simulink model "uc3_preparation1_2017"  (R2018a)
settings: Solver=FixedStepDiscrete  StartTime=0.0  StopTime=0.6  FixedStep=2e-5  RelTol=1e-3
libraries: simulink x10, hdlsllib x10, dspswit3 x1
(part 1 of 2)
settings Model: Creator=elahifah16  LastModifiedBy=Talha Rao
settings OptimizationCC: DefaultParameterBehavior=Inlined  DefaultUnderspecifiedDataType=single  PassReuseOutputArgsAs=Individual arguments
settings DebuggingCC: ParameterTunabilityLossMsg=error  BusObjectLabelMismatch=error
settings HardwareCC: ProdBitPerPointer=32  ProdBitPerSizeT=32  ProdBitPerPtrDiffT=32  ProdLargestAtomicInteger=Long  ProdLargestAtomicFloat=Double  ProdIntDivRoundTo=Undefined  ProdEndianess=Unspecified  ProdWordSize=32  ProdHWDeviceType=ARM Compatible->ARM Cortex
settings SFSimCC: MATLABDynamicMemAlloc=off
settings RTWCC: SystemTargetFile=ert.tlc  GenCodeOnly=on  TemplateMakefile=ert_default_tmf  GenerateReport=on  IncludeHyperlinkInReport=on  LaunchReport=on  GenerateTraceInfo=on  GenerateTraceReport=on  GenerateTraceReportSl=on  GenerateTraceReportSf=on  GenerateTraceReportEml=on  GenerateCodeReplacementReport=on
settings CodeAppCC: ForceParamTrailComments=on  IgnoreCustomStorageClasses=off  OperatorAnnotations=on  SimulinkDataObjDesc=on  SFDataObjDesc=on  InsertBlockDesc=on  StateflowObjectComments=on
settings ERTTargetCC: TargetLangStandard=C99 (ISO)  CodeReplacementLibrary=GNU C99 extensions  GenerateSampleERTMain=on  SupportComplex=off  SupportVariableSizeSignals=on  ExtModeTransport=1  ExtModeMexFile=ext_serial_win32_comm  InlinedParameterPlacement=NonHierarchical  MultiInstanceErrorCode=None  RootIOFormat=Structure reference  ERTCustomFileTemplate=example_file_process.tlc

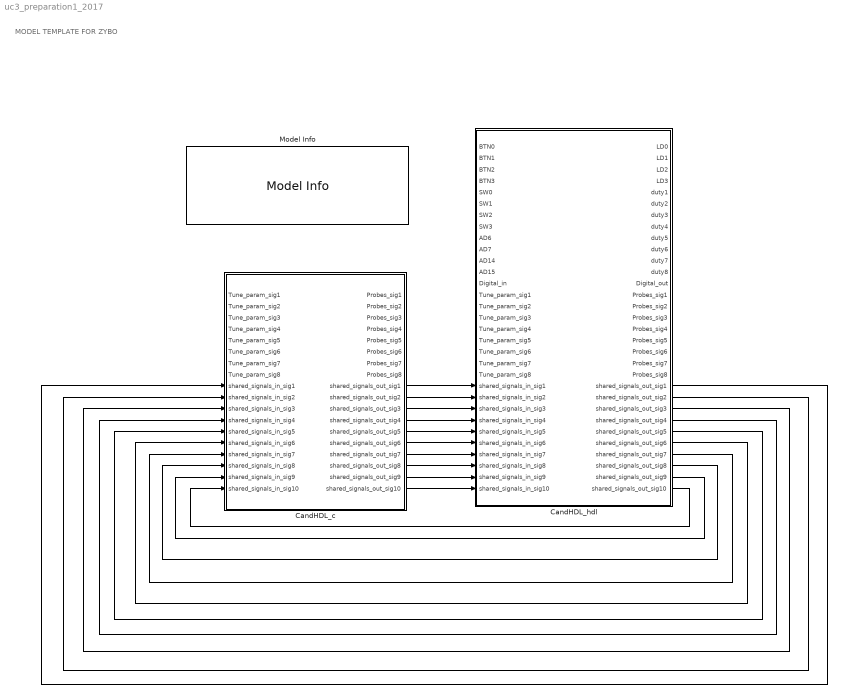
== system uc3_preparation1_2017 ==
  note: MODEL TEMPLATE FOR ZYBO
  CandHDL_c : Subsystem  AncestorBlock=code_gen_library/CandHDL_c
  CandHDL_hdl : Subsystem  AncestorBlock=code_gen_library/CandHDL_hdl
  Model Info : simulink/Model-Wide Utilities/Model Info  Frame=on  DisplayStringWithTags=|  HorizontalTextAlignment=Left  LeftAlignmentValue=0.02
      | Model Info
      | Creator:       R. Estrada, FH JOANNEUM, 2018
      | Modified by: %<ModifiedBy>
      | Modify Date: %<ModifiedDate>
      | Version:%<ModelVersion>
      | Description:
      | %<Description>
  wires:
  CandHDL_c/9(shared_signals_out_sig1) -> CandHDL_hdl/22(shared_signals_in_sig1)
  CandHDL_hdl/22(shared_signals_out_sig1) -> CandHDL_c/9(shared_signals_in_sig1)
  CandHDL_c/10(shared_signals_out_sig2) -> CandHDL_hdl/23(shared_signals_in_sig2)
  CandHDL_hdl/23(shared_signals_out_sig2) -> CandHDL_c/10(shared_signals_in_sig2)
  CandHDL_c/11(shared_signals_out_sig3) -> CandHDL_hdl/24(shared_signals_in_sig3)
  CandHDL_hdl/24(shared_signals_out_sig3) -> CandHDL_c/11(shared_signals_in_sig3)
  CandHDL_c/12(shared_signals_out_sig4) -> CandHDL_hdl/25(shared_signals_in_sig4)
  CandHDL_hdl/25(shared_signals_out_sig4) -> CandHDL_c/12(shared_signals_in_sig4)
  CandHDL_c/13(shared_signals_out_sig5) -> CandHDL_hdl/26(shared_signals_in_sig5)
  CandHDL_hdl/26(shared_signals_out_sig5) -> CandHDL_c/13(shared_signals_in_sig5)
  CandHDL_c/14(shared_signals_out_sig6) -> CandHDL_hdl/27(shared_signals_in_sig6)
  CandHDL_hdl/27(shared_signals_out_sig6) -> CandHDL_c/14(shared_signals_in_sig6)
  CandHDL_c/15(shared_signals_out_sig7) -> CandHDL_hdl/28(shared_signals_in_sig7)
  CandHDL_hdl/28(shared_signals_out_sig7) -> CandHDL_c/15(shared_signals_in_sig7)
  CandHDL_c/16(shared_signals_out_sig8) -> CandHDL_hdl/29(shared_signals_in_sig8)
  CandHDL_hdl/29(shared_signals_out_sig8) -> CandHDL_c/16(shared_signals_in_sig8)
  CandHDL_c/17(shared_signals_out_sig9) -> CandHDL_hdl/30(shared_signals_in_sig9)
  CandHDL_hdl/30(shared_signals_out_sig9) -> CandHDL_c/17(shared_signals_in_sig9)
  CandHDL_c/18(shared_signals_out_sig10) -> CandHDL_hdl/31(shared_signals_in_sig10)
  CandHDL_hdl/31(shared_signals_out_sig10) -> CandHDL_c/18(shared_signals_in_sig10)

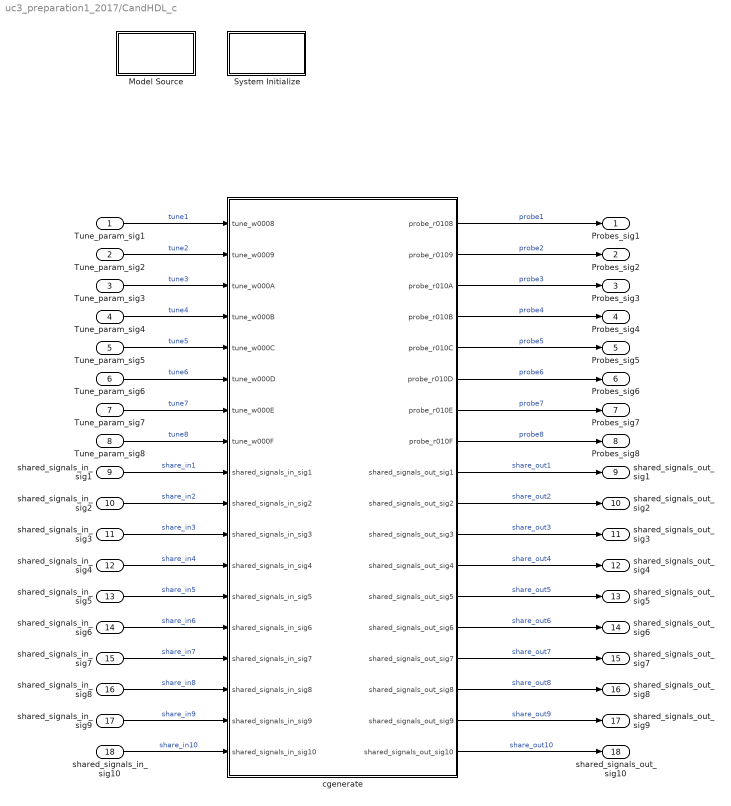
== system uc3_preparation1_2017/CandHDL_c ==
  Tune_param_sig1 : Inport  OutDataTypeStr=int32
  Tune_param_sig2 : Inport  Port=2  OutDataTypeStr=int32
  Tune_param_sig3 : Inport  Port=3  OutDataTypeStr=int32
  Tune_param_sig4 : Inport  Port=4  OutDataTypeStr=int32
  Tune_param_sig5 : Inport  Port=5  OutDataTypeStr=int32
  Tune_param_sig6 : Inport  Port=6  OutDataTypeStr=int32
  Tune_param_sig7 : Inport  Port=7  OutDataTypeStr=int32
  Tune_param_sig8 : Inport  Port=8  OutDataTypeStr=int32
  shared_signals_in_sig1 : Inport  Port=9  OutDataTypeStr=int32
  shared_signals_in_sig2 : Inport  Port=10  OutDataTypeStr=int32
  shared_signals_in_sig3 : Inport  Port=11  OutDataTypeStr=int32
  shared_signals_in_sig4 : Inport  Port=12  OutDataTypeStr=int32
  shared_signals_in_sig5 : Inport  Port=13  OutDataTypeStr=int32
  shared_signals_in_sig6 : Inport  Port=14  OutDataTypeStr=int32
  shared_signals_in_sig7 : Inport  Port=15  OutDataTypeStr=int32
  shared_signals_in_sig8 : Inport  Port=16  OutDataTypeStr=int32
  shared_signals_in_sig9 : Inport  Port=17  OutDataTypeStr=int32
  shared_signals_in_sig10 : Inport  Port=18  OutDataTypeStr=int32
  Model Source : Subsystem  mask(Model Source){ShowInLibBrowser=0}
      mask prompts: ShowInLibBrowser "Simulink:masks:CustCodeMaskParam1_MP"
      settings: CopyFcn=cccopyfcn(gcb)  OpenFcn=ccopenfcn('Model Source')
      mask Help: eval('feval(''rtwprivate'',''rtwhelpview'',''rtw_model_source_block'')');
      mask Display: disp('Model\nSource');
  System Initialize : Subsystem  mask(System Initialize){ShowInLibBrowser=0}
      mask prompts: ShowInLibBrowser "Simulink:masks:CustCodeMaskParam1_MP"
      settings: CopyFcn=cccopyfcn(gcb)  OpenFcn=ccopenfcn('System Initialize Function')
      mask Help: eval('feval(''rtwprivate'',''rtwhelpview'',''rtw_sys_initialize_block'')');
      mask Display: disp('System\nInitialize');
  cgenerate : Subsystem
  Probes_sig1 : Outport  OutDataTypeStr=int32
  Probes_sig2 : Outport  Port=2  OutDataTypeStr=int32
  Probes_sig3 : Outport  Port=3  OutDataTypeStr=int32
  Probes_sig4 : Outport  Port=4  OutDataTypeStr=int32
  Probes_sig5 : Outport  Port=5  OutDataTypeStr=int32
  Probes_sig6 : Outport  Port=6  OutDataTypeStr=int32
  Probes_sig7 : Outport  Port=7  OutDataTypeStr=int32
  Probes_sig8 : Outport  Port=8  OutDataTypeStr=int32
  shared_signals_out_sig1 : Outport  Port=9  OutDataTypeStr=int32
  shared_signals_out_sig2 : Outport  Port=10  OutDataTypeStr=int32
  shared_signals_out_sig3 : Outport  Port=11  OutDataTypeStr=int32
  shared_signals_out_sig4 : Outport  Port=12  OutDataTypeStr=int32
  shared_signals_out_sig5 : Outport  Port=13  OutDataTypeStr=int32
  shared_signals_out_sig6 : Outport  Port=14  OutDataTypeStr=int32
  shared_signals_out_sig7 : Outport  Port=15  OutDataTypeStr=int32
  shared_signals_out_sig8 : Outport  Port=16  OutDataTypeStr=int32
  shared_signals_out_sig9 : Outport  Port=17  OutDataTypeStr=int32
  shared_signals_out_sig10 : Outport  Port=18  OutDataTypeStr=int32
  wires:
  cgenerate/1(probe_r0108) -> Probes_sig1/1  "probe1"
  cgenerate/2(probe_r0109) -> Probes_sig2/1  "probe2"
  cgenerate/3(probe_r010A) -> Probes_sig3/1  "probe3"
  cgenerate/4(probe_r010B) -> Probes_sig4/1  "probe4"
  cgenerate/5(probe_r010C) -> Probes_sig5/1  "probe5"
  cgenerate/6(probe_r010D) -> Probes_sig6/1  "probe6"
  cgenerate/7(probe_r010E) -> Probes_sig7/1  "probe7"
  cgenerate/8(probe_r010F) -> Probes_sig8/1  "probe8"
  Tune_param_sig1/1 -> cgenerate/1(tune_w0008)  "tune1"
  Tune_param_sig2/1 -> cgenerate/2(tune_w0009)  "tune2"
  Tune_param_sig3/1 -> cgenerate/3(tune_w000A)  "tune3"
  Tune_param_sig4/1 -> cgenerate/4(tune_w000B)  "tune4"
  Tune_param_sig5/1 -> cgenerate/5(tune_w000C)  "tune5"
  Tune_param_sig6/1 -> cgenerate/6(tune_w000D)  "tune6"
  Tune_param_sig7/1 -> cgenerate/7(tune_w000E)  "tune7"
  Tune_param_sig8/1 -> cgenerate/8(tune_w000F)  "tune8"
  shared_signals_in_sig1/1 -> cgenerate/9(shared_signals_in_sig1)  "share_in1"
  shared_signals_in_sig2/1 -> cgenerate/10(shared_signals_in_sig2)  "share_in2"
  shared_signals_in_sig3/1 -> cgenerate/11(shared_signals_in_sig3)  "share_in3"
  shared_signals_in_sig4/1 -> cgenerate/12(shared_signals_in_sig4)  "share_in4"
  shared_signals_in_sig5/1 -> cgenerate/13(shared_signals_in_sig5)  "share_in5"
  shared_signals_in_sig6/1 -> cgenerate/14(shared_signals_in_sig6)  "share_in6"
  shared_signals_in_sig7/1 -> cgenerate/15(shared_signals_in_sig7)  "share_in7"
  shared_signals_in_sig8/1 -> cgenerate/16(shared_signals_in_sig8)  "share_in8"
  shared_signals_in_sig9/1 -> cgenerate/17(shared_signals_in_sig9)  "share_in9"
  shared_signals_in_sig10/1 -> cgenerate/18(shared_signals_in_sig10)  "share_in10"
  cgenerate/9(shared_signals_out_sig1) -> shared_signals_out_sig1/1  "share_out1"
  cgenerate/10(shared_signals_out_sig2) -> shared_signals_out_sig2/1  "share_out2"
  cgenerate/11(shared_signals_out_sig3) -> shared_signals_out_sig3/1  "share_out3"
  cgenerate/12(shared_signals_out_sig4) -> shared_signals_out_sig4/1  "share_out4"
  cgenerate/13(shared_signals_out_sig5) -> shared_signals_out_sig5/1  "share_out5"
  cgenerate/14(shared_signals_out_sig6) -> shared_signals_out_sig6/1  "share_out6"
  cgenerate/15(shared_signals_out_sig7) -> shared_signals_out_sig7/1  "share_out7"
  cgenerate/16(shared_signals_out_sig8) -> shared_signals_out_sig8/1  "share_out8"
  cgenerate/17(shared_signals_out_sig9) -> shared_signals_out_sig9/1  "share_out9"
  cgenerate/18(shared_signals_out_sig10) -> shared_signals_out_sig10/1  "share_out10"

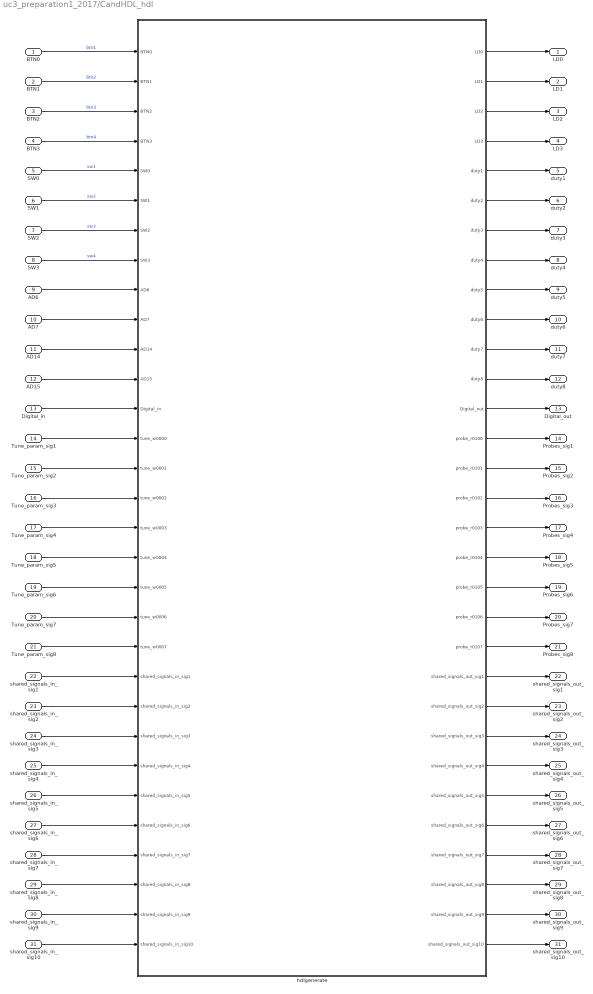
== system uc3_preparation1_2017/CandHDL_hdl ==
  BTN0 : Inport  OutDataTypeStr=boolean
  BTN1 : Inport  Port=2  OutDataTypeStr=boolean
  BTN2 : Inport  Port=3  OutDataTypeStr=boolean
  BTN3 : Inport  Port=4  OutDataTypeStr=boolean
  SW0 : Inport  Port=5  OutDataTypeStr=boolean
  SW1 : Inport  Port=6  OutDataTypeStr=boolean
  SW2 : Inport  Port=7  OutDataTypeStr=boolean
  SW3 : Inport  Port=8  OutDataTypeStr=boolean
  AD6 : Inport  Port=9  OutDataTypeStr=uint16
  AD7 : Inport  Port=10  OutDataTypeStr=uint16
  AD14 : Inport  Port=11  OutDataTypeStr=uint16
  AD15 : Inport  Port=12  OutDataTypeStr=uint16
  Digital_in : Inport  Port=13  OutDataTypeStr=uint8
  Tune_param_sig1 : Inport  Port=14  OutDataTypeStr=int32
  Tune_param_sig2 : Inport  Port=15  OutDataTypeStr=int32
  Tune_param_sig3 : Inport  Port=16  OutDataTypeStr=int32
  Tune_param_sig4 : Inport  Port=17  OutDataTypeStr=int32
  Tune_param_sig5 : Inport  Port=18  OutDataTypeStr=int32
  Tune_param_sig6 : Inport  Port=19  OutDataTypeStr=int32
  Tune_param_sig7 : Inport  Port=20  OutDataTypeStr=int32
  Tune_param_sig8 : Inport  Port=21  OutDataTypeStr=int32
  shared_signals_in_sig1 : Inport  Port=22  OutDataTypeStr=int32
  shared_signals_in_sig2 : Inport  Port=23  OutDataTypeStr=int32
  shared_signals_in_sig3 : Inport  Port=24  OutDataTypeStr=int32
  shared_signals_in_sig4 : Inport  Port=25  OutDataTypeStr=int32
  shared_signals_in_sig5 : Inport  Port=26  OutDataTypeStr=int32
  shared_signals_in_sig6 : Inport  Port=27  OutDataTypeStr=int32
  shared_signals_in_sig7 : Inport  Port=28  OutDataTypeStr=int32
  shared_signals_in_sig8 : Inport  Port=29  OutDataTypeStr=int32
  shared_signals_in_sig9 : Inport  Port=30  OutDataTypeStr=int32
  shared_signals_in_sig10 : Inport  Port=31  OutDataTypeStr=int32
  hdlgenerate : Subsystem
  LD0 : Outport  OutDataTypeStr=boolean
  LD1 : Outport  Port=2  OutDataTypeStr=boolean
  LD2 : Outport  Port=3  OutDataTypeStr=boolean
  LD3 : Outport  Port=4  OutDataTypeStr=boolean
  duty1 : Outport  Port=5  OutDataTypeStr=uint16
  duty2 : Outport  Port=6  OutDataTypeStr=uint16
  duty3 : Outport  Port=7  OutDataTypeStr=uint16
  duty4 : Outport  Port=8  OutDataTypeStr=uint16
  duty5 : Outport  Port=9  OutDataTypeStr=uint16
  duty6 : Outport  Port=10  OutDataTypeStr=uint16
  duty7 : Outport  Port=11  OutDataTypeStr=uint16
  duty8 : Outport  Port=12  OutDataTypeStr=uint16
  Digital_out : Outport  Port=13  OutDataTypeStr=uint8
  Probes_sig1 : Outport  Port=14  OutDataTypeStr=int32
  Probes_sig2 : Outport  Port=15  OutDataTypeStr=int32
  Probes_sig3 : Outport  Port=16  OutDataTypeStr=int32
  Probes_sig4 : Outport  Port=17  OutDataTypeStr=int32
  Probes_sig5 : Outport  Port=18  OutDataTypeStr=int32
  Probes_sig6 : Outport  Port=19  OutDataTypeStr=int32
  Probes_sig7 : Outport  Port=20  OutDataTypeStr=int32
  Probes_sig8 : Outport  Port=21  OutDataTypeStr=int32
  shared_signals_out_sig1 : Outport  Port=22  OutDataTypeStr=int32
  shared_signals_out_sig2 : Outport  Port=23  OutDataTypeStr=int32
  shared_signals_out_sig3 : Outport  Port=24  OutDataTypeStr=int32
  shared_signals_out_sig4 : Outport  Port=25  OutDataTypeStr=int32
  shared_signals_out_sig5 : Outport  Port=26  OutDataTypeStr=int32
  shared_signals_out_sig6 : Outport  Port=27  OutDataTypeStr=int32
  shared_signals_out_sig7 : Outport  Port=28  OutDataTypeStr=int32
  shared_signals_out_sig8 : Outport  Port=29  OutDataTypeStr=int32
  shared_signals_out_sig9 : Outport  Port=30  OutDataTypeStr=int32
  shared_signals_out_sig10 : Outport  Port=31  OutDataTypeStr=int32
  wires:
  hdlgenerate/1(LD0) -> LD0/1
  hdlgenerate/2(LD1) -> LD1/1
  hdlgenerate/3(LD2) -> LD2/1
  hdlgenerate/4(LD3) -> LD3/1
  hdlgenerate/5(duty1) -> duty1/1
  hdlgenerate/6(duty2) -> duty2/1
  hdlgenerate/7(duty3) -> duty3/1
  hdlgenerate/8(duty4) -> duty4/1
  hdlgenerate/9(duty5) -> duty5/1
  hdlgenerate/10(duty6) -> duty6/1
  hdlgenerate/11(duty7) -> duty7/1
  hdlgenerate/12(duty8) -> duty8/1
  hdlgenerate/13(Digital_out) -> Digital_out/1
  hdlgenerate/14(probe_r0100) -> Probes_sig1/1
  hdlgenerate/15(probe_r0101) -> Probes_sig2/1
  hdlgenerate/16(probe_r0102) -> Probes_sig3/1
  hdlgenerate/17(probe_r0103) -> Probes_sig4/1
  hdlgenerate/18(probe_r0104) -> Probes_sig5/1
  hdlgenerate/19(probe_r0105) -> Probes_sig6/1
  hdlgenerate/20(probe_r0106) -> Probes_sig7/1
  hdlgenerate/21(probe_r0107) -> Probes_sig8/1
  hdlgenerate/22(shared_signals_out_sig1) -> shared_signals_out_sig1/1
  hdlgenerate/23(shared_signals_out_sig2) -> shared_signals_out_sig2/1
  hdlgenerate/24(shared_signals_out_sig3) -> shared_signals_out_sig3/1
  hdlgenerate/25(shared_signals_out_sig4) -> shared_signals_out_sig4/1
  hdlgenerate/26(shared_signals_out_sig5) -> shared_signals_out_sig5/1
  hdlgenerate/27(shared_signals_out_sig6) -> shared_signals_out_sig6/1
  hdlgenerate/28(shared_signals_out_sig7) -> shared_signals_out_sig7/1
  hdlgenerate/29(shared_signals_out_sig8) -> shared_signals_out_sig8/1
  hdlgenerate/30(shared_signals_out_sig9) -> shared_signals_out_sig9/1
  hdlgenerate/31(shared_signals_out_sig10) -> shared_signals_out_sig10/1
  BTN0/1 -> hdlgenerate/1(BTN0)  "btn1"
  BTN1/1 -> hdlgenerate/2(BTN1)  "btn2"
  BTN2/1 -> hdlgenerate/3(BTN2)  "btn3"
  BTN3/1 -> hdlgenerate/4(BTN3)  "btn4"
  SW0/1 -> hdlgenerate/5(SW0)  "sw1"
  SW1/1 -> hdlgenerate/6(SW1)  "sw2"
  SW2/1 -> hdlgenerate/7(SW2)  "sw3"
  SW3/1 -> hdlgenerate/8(SW3)  "sw4"
  AD6/1 -> hdlgenerate/9(AD6)
  AD7/1 -> hdlgenerate/10(AD7)
  AD14/1 -> hdlgenerate/11(AD14)
  AD15/1 -> hdlgenerate/12(AD15)
  Digital_in/1 -> hdlgenerate/13(Digital_in)
  Tune_param_sig1/1 -> hdlgenerate/14(tune_w0000)
  Tune_param_sig2/1 -> hdlgenerate/15(tune_w0001)
  Tune_param_sig3/1 -> hdlgenerate/16(tune_w0002)
  Tune_param_sig4/1 -> hdlgenerate/17(tune_w0003)
  Tune_param_sig5/1 -> hdlgenerate/18(tune_w0004)
  Tune_param_sig6/1 -> hdlgenerate/19(tune_w0005)
  Tune_param_sig7/1 -> hdlgenerate/20(tune_w0006)
  Tune_param_sig8/1 -> hdlgenerate/21(tune_w0007)
  shared_signals_in_sig1/1 -> hdlgenerate/22(shared_signals_in_sig1)
  shared_signals_in_sig2/1 -> hdlgenerate/23(shared_signals_in_sig2)
  shared_signals_in_sig3/1 -> hdlgenerate/24(shared_signals_in_sig3)
  shared_signals_in_sig4/1 -> hdlgenerate/25(shared_signals_in_sig4)
  shared_signals_in_sig5/1 -> hdlgenerate/26(shared_signals_in_sig5)
  shared_signals_in_sig6/1 -> hdlgenerate/27(shared_signals_in_sig6)
  shared_signals_in_sig7/1 -> hdlgenerate/28(shared_signals_in_sig7)
  shared_signals_in_sig8/1 -> hdlgenerate/29(shared_signals_in_sig8)
  shared_signals_in_sig9/1 -> hdlgenerate/30(shared_signals_in_sig9)
  shared_signals_in_sig10/1 -> hdlgenerate/31(shared_signals_in_sig10)

== system uc3_preparation1_2017/CandHDL_c/Model Source ==

== system uc3_preparation1_2017/CandHDL_c/System Initialize ==

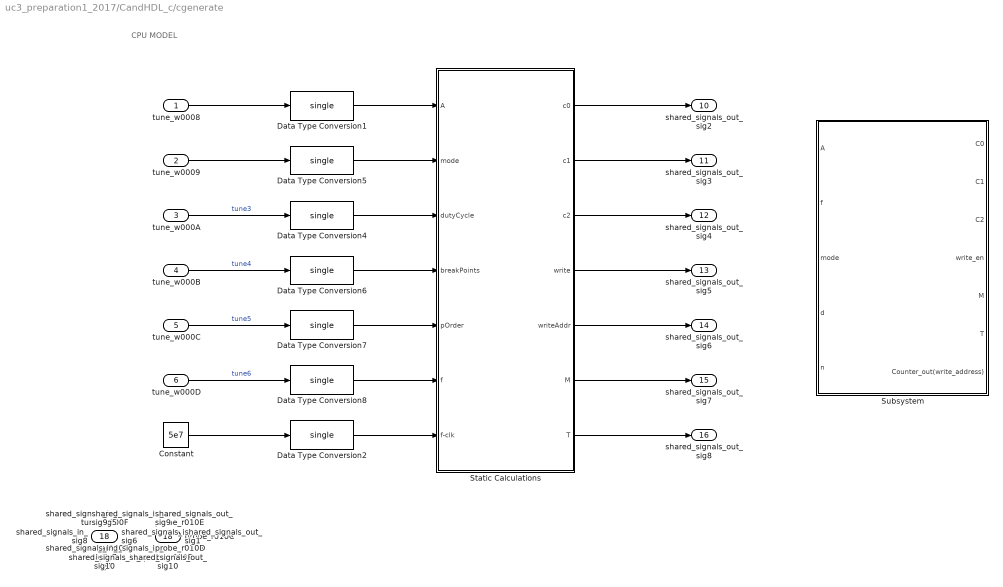
== system uc3_preparation1_2017/CandHDL_c/cgenerate ==
  note: CPU MODEL
  tune_w0008 : Inport  OutDataTypeStr=int32
  tune_w0009 : Inport  Port=2  OutDataTypeStr=int32
  tune_w000A : Inport  Port=3  OutDataTypeStr=int32
  tune_w000B : Inport  Port=4  OutDataTypeStr=int32
  tune_w000C : Inport  Port=5  OutDataTypeStr=int32
  tune_w000D : Inport  Port=6  OutDataTypeStr=int32
  tune_w000E : Inport  Port=7  OutDataTypeStr=int32
  tune_w000F : Inport  Port=8  OutDataTypeStr=int32
  shared_signals_in_sig1 : Inport  Port=9  OutDataTypeStr=int32
  shared_signals_in_sig2 : Inport  Port=10  OutDataTypeStr=int32
  shared_signals_in_sig3 : Inport  Port=11  OutDataTypeStr=int32
  shared_signals_in_sig4 : Inport  Port=12  OutDataTypeStr=int32
  shared_signals_in_sig5 : Inport  Port=13  OutDataTypeStr=int32
  shared_signals_in_sig6 : Inport  Port=14  OutDataTypeStr=int32
  shared_signals_in_sig7 : Inport  Port=15  OutDataTypeStr=int32
  shared_signals_in_sig8 : Inport  Port=16  OutDataTypeStr=int32
  shared_signals_in_sig9 : Inport  Port=17  OutDataTypeStr=int32
  shared_signals_in_sig10 : Inport  Port=18  OutDataTypeStr=int32
  Constant : Constant  Value=5e7
  Data Type Conversion{1..2,4..8} (7 alike) : DataTypeConversion  OutDataTypeStr=single
  Static Calculations : Subsystem
  Subsystem : Subsystem
  probe_r0108 : Outport  OutDataTypeStr=int32
  probe_r0109 : Outport  Port=2  OutDataTypeStr=int32
  probe_r010A : Outport  Port=3  OutDataTypeStr=int32
  probe_r010B : Outport  Port=4  OutDataTypeStr=int32
  probe_r010C : Outport  Port=5  OutDataTypeStr=int32
  probe_r010D : Outport  Port=6  OutDataTypeStr=int32
  probe_r010E : Outport  Port=7  OutDataTypeStr=int32
  probe_r010F : Outport  Port=8  OutDataTypeStr=int32
  shared_signals_out_sig1 : Outport  Port=9  OutDataTypeStr=int32
  shared_signals_out_sig2 : Outport  Port=10  OutDataTypeStr=int32
  shared_signals_out_sig3 : Outport  Port=11  OutDataTypeStr=int32
  shared_signals_out_sig4 : Outport  Port=12  OutDataTypeStr=int32
  shared_signals_out_sig5 : Outport  Port=13  OutDataTypeStr=int32
  shared_signals_out_sig6 : Outport  Port=14  OutDataTypeStr=int32
  shared_signals_out_sig7 : Outport  Port=15  OutDataTypeStr=int32
  shared_signals_out_sig8 : Outport  Port=16  OutDataTypeStr=int32
  shared_signals_out_sig9 : Outport  Port=17  OutDataTypeStr=int32
  shared_signals_out_sig10 : Outport  Port=18  OutDataTypeStr=int32
  wires:
  tune_w000C/1 -> Data Type Conversion7/1  "tune5"
  tune_w0008/1 -> Data Type Conversion1/1
  tune_w0009/1 -> Data Type Conversion5/1
  tune_w000A/1 -> Data Type Conversion4/1  "tune3"
  tune_w000B/1 -> Data Type Conversion6/1  "tune4"
  Static Calculations/1(c0) -> shared_signals_out_sig2/1
  Static Calculations/5(writeAddr) -> shared_signals_out_sig6/1
  Static Calculations/2(c1) -> shared_signals_out_sig3/1
  Static Calculations/3(c2) -> shared_signals_out_sig4/1
  Static Calculations/4(write) -> shared_signals_out_sig5/1
  Static Calculations/6(M) -> shared_signals_out_sig7/1
  Static Calculations/7(T) -> shared_signals_out_sig8/1
  Data Type Conversion1/1 -> Static Calculations/1(A)
  Data Type Conversion5/1 -> Static Calculations/2(mode)
  Data Type Conversion4/1 -> Static Calculations/3(dutyCycle)
  Data Type Conversion6/1 -> Static Calculations/4(breakPoints)
  Data Type Conversion7/1 -> Static Calculations/5(pOrder)
  tune_w000D/1 -> Data Type Conversion8/1  "tune6"
  Data Type Conversion8/1 -> Static Calculations/6(f)
  Constant/1 -> Data Type Conversion2/1
  Data Type Conversion2/1 -> Static Calculations/7(f-clk)

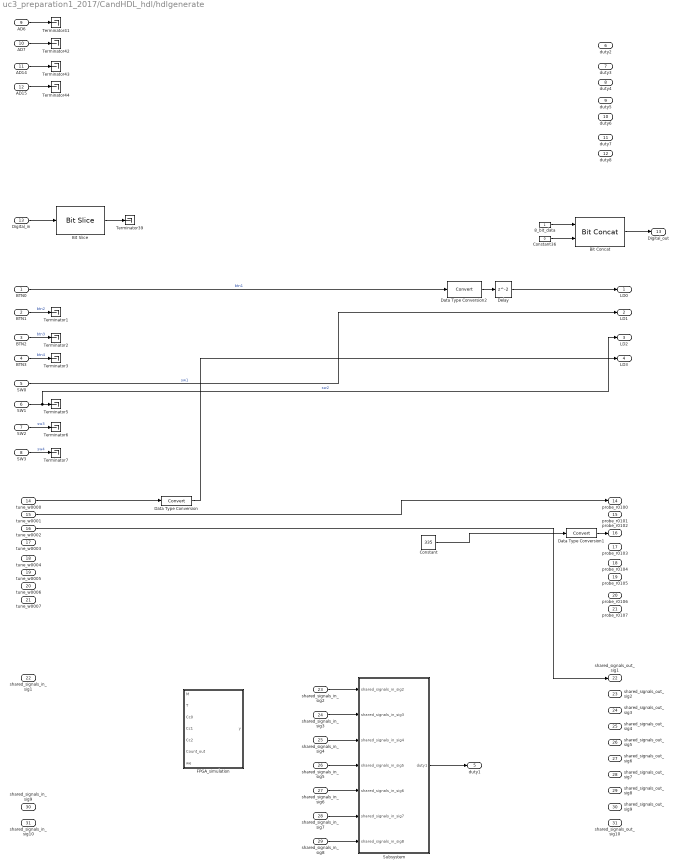
== system uc3_preparation1_2017/CandHDL_hdl/hdlgenerate ==
  BTN0 : Inport  OutDataTypeStr=boolean
  BTN1 : Inport  Port=2  OutDataTypeStr=boolean
  BTN2 : Inport  Port=3  OutDataTypeStr=boolean
  BTN3 : Inport  Port=4  OutDataTypeStr=boolean
  SW0 : Inport  Port=5  OutDataTypeStr=boolean
  SW1 : Inport  Port=6  OutDataTypeStr=boolean
  SW2 : Inport  Port=7  OutDataTypeStr=boolean
  SW3 : Inport  Port=8  OutDataTypeStr=boolean
  AD6 : Inport  Port=9  OutDataTypeStr=uint16
  AD7 : Inport  Port=10  OutDataTypeStr=uint16
  AD14 : Inport  Port=11  OutDataTypeStr=uint16
  AD15 : Inport  Port=12  OutDataTypeStr=uint16
  Digital_in : Inport  Port=13  OutDataTypeStr=uint8
  tune_w0000 : Inport  Port=14  OutDataTypeStr=int32
  tune_w0001 : Inport  Port=15  OutDataTypeStr=int32
  tune_w0002 : Inport  Port=16  OutDataTypeStr=int32
  tune_w0003 : Inport  Port=17  OutDataTypeStr=int32
  tune_w0004 : Inport  Port=18  OutDataTypeStr=int32
  tune_w0005 : Inport  Port=19  OutDataTypeStr=int32
  tune_w0006 : Inport  Port=20  OutDataTypeStr=int32
  tune_w0007 : Inport  Port=21  OutDataTypeStr=int32
  shared_signals_in_sig1 : Inport  Port=22  OutDataTypeStr=int32
  shared_signals_in_sig2 : Inport  Port=23  OutDataTypeStr=int32
  shared_signals_in_sig3 : Inport  Port=24  OutDataTypeStr=int32
  shared_signals_in_sig4 : Inport  Port=25  OutDataTypeStr=int32
  shared_signals_in_sig5 : Inport  Port=26  OutDataTypeStr=int32
  shared_signals_in_sig6 : Inport  Port=27  OutDataTypeStr=int32
  shared_signals_in_sig7 : Inport  Port=28  OutDataTypeStr=int32
  shared_signals_in_sig8 : Inport  Port=29  OutDataTypeStr=int32
  shared_signals_in_sig9 : Inport  Port=30  OutDataTypeStr=int32
  shared_signals_in_sig10 : Inport  Port=31  OutDataTypeStr=int32
  8_bit_data : Constant  OutDataTypeStr=fixdt(0,4,0)  SampleTime=-1
  Bit Concat : hdlsllib/Logic and Bit Operations/Bit Concat  numInputs=2
      settings: SourceProductName=HDL Coder  SourceProductBaseCode=HD
  Bit Slice : hdlsllib/Logic and Bit Operations/Bit Slice  lidx=0  ridx=0
  Constant : Constant  Value=335  OutDataTypeStr=int16  SampleTime=-1
  Constant36 : Constant  Value=0  OutDataTypeStr=fixdt(0,4,0)  SampleTime=-1
  Data Type Conversion : DataTypeConversion
  Data Type Conversion1 : DataTypeConversion
  Data Type Conversion2 : DataTypeConversion
  Delay : Delay
  FPGA_simulation : Subsystem
  Subsystem : Subsystem
  Terminator{1..3,5..7,39,41..44} (11 alike) : Terminator
  LD0 : Outport  OutDataTypeStr=boolean
  LD1 : Outport  Port=2  OutDataTypeStr=boolean
  LD2 : Outport  Port=3  OutDataTypeStr=boolean
  LD3 : Outport  Port=4  OutDataTypeStr=boolean
  duty1 : Outport  Port=5  OutDataTypeStr=uint16
  duty2 : Outport  Port=6  OutDataTypeStr=uint16
  duty3 : Outport  Port=7  OutDataTypeStr=uint16
  duty4 : Outport  Port=8  OutDataTypeStr=uint16
  duty5 : Outport  Port=9  OutDataTypeStr=uint16
  duty6 : Outport  Port=10  OutDataTypeStr=uint16
  duty7 : Outport  Port=11  OutDataTypeStr=uint16
  duty8 : Outport  Port=12  OutDataTypeStr=uint16
  Digital_out : Outport  Port=13  OutDataTypeStr=uint8
  probe_r0100 : Outport  Port=14  OutDataTypeStr=int32
  probe_r0101 : Outport  Port=15  OutDataTypeStr=int32
  probe_r0102 : Outport  Port=16  OutDataTypeStr=int32
  probe_r0103 : Outport  Port=17  OutDataTypeStr=int32
  probe_r0104 : Outport  Port=18  OutDataTypeStr=int32
  probe_r0105 : Outport  Port=19  OutDataTypeStr=int32
  probe_r0106 : Outport  Port=20  OutDataTypeStr=int32
  probe_r0107 : Outport  Port=21  OutDataTypeStr=int32
  shared_signals_out_sig1 : Outport  Port=22  OutDataTypeStr=int32
  shared_signals_out_sig2 : Outport  Port=23  OutDataTypeStr=int32
  shared_signals_out_sig3 : Outport  Port=24  OutDataTypeStr=int32
  shared_signals_out_sig4 : Outport  Port=25  OutDataTypeStr=int32
  shared_signals_out_sig5 : Outport  Port=26  OutDataTypeStr=int32
  shared_signals_out_sig6 : Outport  Port=27  OutDataTypeStr=int32
  shared_signals_out_sig7 : Outport  Port=28  OutDataTypeStr=int32
  shared_signals_out_sig8 : Outport  Port=29  OutDataTypeStr=int32
  shared_signals_out_sig9 : Outport  Port=30  OutDataTypeStr=int32
  shared_signals_out_sig10 : Outport  Port=31  OutDataTypeStr=int32
  wires:
  Digital_in/1 -> Bit Slice/1
  Data Type Conversion2/1 -> Delay/1
  AD7/1 -> Terminator42/1
  SW2/1 -> Terminator6/1  "sw3"
  Constant36/1 -> Bit Concat/2
  Data Type Conversion/1 -> LD3/1
  tune_w0001/1 -> probe_r0100/1
  Data Type Conversion1/1 -> probe_r0102/1
  BTN1/1 -> Terminator1/1  "btn2"
  tune_w0002/1 -> shared_signals_out_sig1/1
  tune_w0000/1 -> Data Type Conversion/1
  SW3/1 -> Terminator7/1  "sw4"
  8_bit_data/1 -> Bit Concat/1
  SW0/1 -> LD1/1  "sw1"
  BTN3/1 -> Terminator3/1  "btn4"
  AD14/1 -> Terminator43/1
  BTN2/1 -> Terminator2/1  "btn3"
  Bit Slice/1 -> Terminator39/1
  Constant/1 -> Data Type Conversion1/1
  SW1/1 -> LD2/1, Terminator5/1  "sw2"
  Bit Concat/1 -> Digital_out/1
  AD15/1 -> Terminator44/1
  Delay/1 -> LD0/1
  AD6/1 -> Terminator41/1
  BTN0/1 -> Data Type Conversion2/1  "btn1"
  shared_signals_in_sig2/1 -> Subsystem/1(shared_signals_in_sig2)
  shared_signals_in_sig3/1 -> Subsystem/2(shared_signals_in_sig3)
  shared_signals_in_sig4/1 -> Subsystem/3(shared_signals_in_sig4)
  shared_signals_in_sig5/1 -> Subsystem/4(shared_signals_in_sig5)
  shared_signals_in_sig6/1 -> Subsystem/5(shared_signals_in_sig6)
  shared_signals_in_sig7/1 -> Subsystem/6(shared_signals_in_sig7)
  shared_signals_in_sig8/1 -> Subsystem/7(shared_signals_in_sig8)
  Subsystem/1(duty1) -> duty1/1

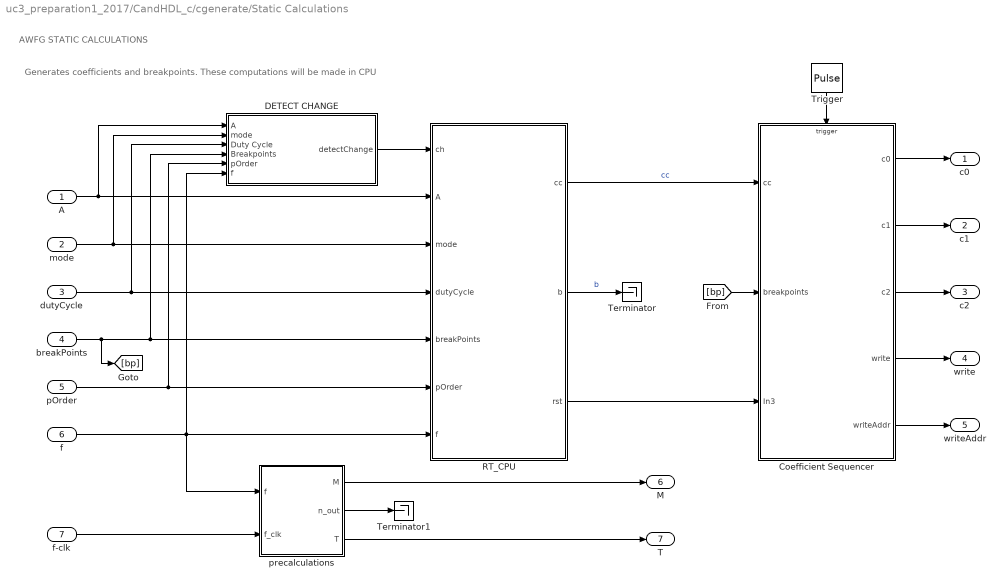
== system uc3_preparation1_2017/CandHDL_c/cgenerate/Static Calculations ==
  note: AWFG STATIC CALCULATIONS
  note: Generates coefficients and breakpoints. These computations will be made in CPU
  A : Inport
  mode : Inport  Port=2
  dutyCycle : Inport  Port=3
  breakPoints : Inport  Port=4
  pOrder : Inport  Port=5
  f : Inport  Port=6
  f-clk : Inport  Port=7
  Coefficient Sequencer : Subsystem
  DETECT CHANGE : Subsystem
  RT_CPU : MATLAB Function  TreatAsAtomicUnit=on
  Terminator : Terminator
  Terminator1 : Terminator
  Trigger : DiscretePulseGenerator  PulseType=Time based  Period=1/5e7  PulseWidth=50
  precalculations : Subsystem
  c0 : Outport
  c1 : Outport  Port=2
  c2 : Outport  Port=3
  write : Outport  Port=4
  writeAddr : Outport  Port=5
  M : Outport  Port=6
  T : Outport  Port=7
  wires:
  RT_CPU/1(cc) -> Coefficient Sequencer/1(cc)  "cc"
  f/1 -> precalculations/1(f), RT_CPU/7(f), DETECT CHANGE/6(f)
  breakPoints/1 -> [bp], DETECT CHANGE/4(Breakpoints), RT_CPU/5(breakPoints)
  f-clk/1 -> precalculations/2(f_clk)
  A/1 -> DETECT CHANGE/1(A), RT_CPU/2(A)
  pOrder/1 -> DETECT CHANGE/5(pOrder), RT_CPU/6(pOrder)
  precalculations/2(n_out) -> Terminator1/1
  mode/1 -> RT_CPU/3(mode), DETECT CHANGE/2(mode)
  dutyCycle/1 -> DETECT CHANGE/3(Duty Cycle), RT_CPU/4(dutyCycle)
  DETECT CHANGE/1(detectChange) -> RT_CPU/1(ch)
  precalculations/3(T) -> T/1
  precalculations/1(M) -> M/1
  Trigger/1 -> Coefficient Sequencer/Trigger
  RT_CPU/3(rst) -> Coefficient Sequencer/3(In3)
  [bp] -> Coefficient Sequencer/2(breakpoints)
  Coefficient Sequencer/1(c0) -> c0/1
  Coefficient Sequencer/2(c1) -> c1/1
  Coefficient Sequencer/3(c2) -> c2/1
  Coefficient Sequencer/4(write) -> write/1
  Coefficient Sequencer/5(writeAddr) -> writeAddr/1
  RT_CPU/2(b) -> Terminator/1  "b"

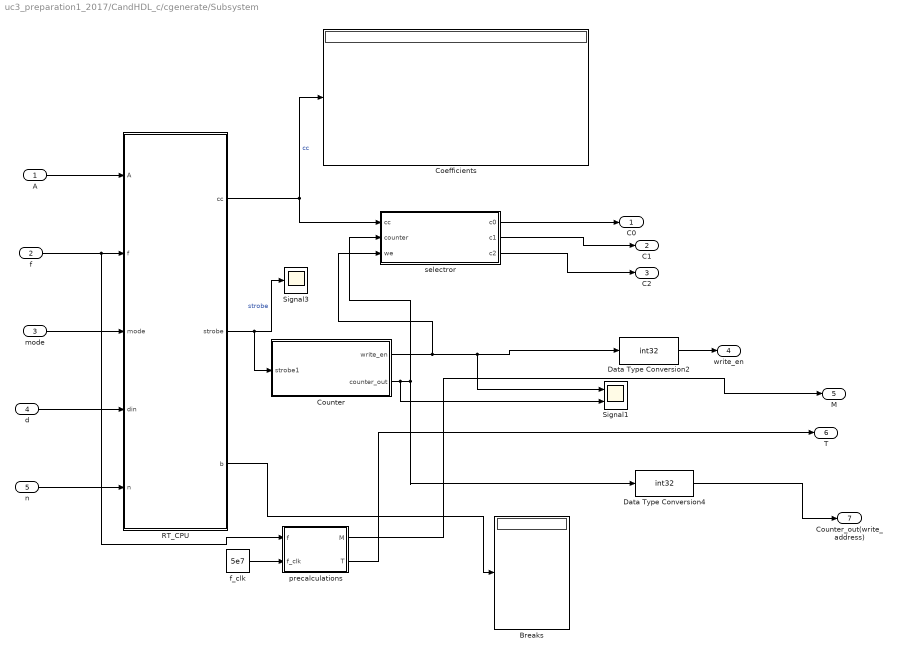
== system uc3_preparation1_2017/CandHDL_c/cgenerate/Subsystem ==
  A : Inport  OutDataTypeStr=single
  "f " : Inport  Port=2  OutDataTypeStr=single
  mode : Inport  Port=3  OutDataTypeStr=single
  d : Inport  Port=4  OutDataTypeStr=single
  n : Inport  Port=5  OutDataTypeStr=single
  Breaks : Display
  Coefficients : Display
  Counter : Subsystem  TreatAsAtomicUnit=on
  Data Type Conversion2 : DataTypeConversion  OutDataTypeStr=int32
  Data Type Conversion4 : DataTypeConversion  OutDataTypeStr=int32
  RT_CPU : MATLAB Function  TreatAsAtomicUnit=on
  Signal1 : Scope  NumInputPorts=2
  Signal3 : Scope
  f_clk : Constant  Value=5e7  OutDataTypeStr=int32
  precalculations : Subsystem
  selectror : Subsystem  TreatAsAtomicUnit=on
  C0 : Outport  OutDataTypeStr=int32
  C1 : Outport  Port=2  OutDataTypeStr=int32
  C2 : Outport  Port=3  OutDataTypeStr=int32
  write_en : Outport  Port=4  OutDataTypeStr=int32
  M : Outport  Port=5  OutDataTypeStr=int32
  T : Outport  Port=6  OutDataTypeStr=int32
  Counter_out(write_address) : Outport  Port=7  OutDataTypeStr=int32
  wires:
  selectror/2(c1) -> C1/1
  Data Type Conversion2/1 -> write_en/1
  precalculations/1(M) -> M/1
  precalculations/2(T) -> T/1
  selectror/1(c0) -> C0/1
  selectror/3(c2) -> C2/1
  A/1 -> RT_CPU/1(A)
  Counter/1(write_en) -> selectror/3(we), Signal1/1, Data Type Conversion2/1
  "f "/1 -> precalculations/1(f), RT_CPU/2(f)
  RT_CPU/1(cc) -> selectror/1(cc), Coefficients/1  "cc"
  Counter/2(counter_out) -> selectror/2(counter), Data Type Conversion4/1, Signal1/2
  n/1 -> RT_CPU/5(n)
  RT_CPU/2(strobe) -> Counter/1(strobe1), Signal3/1  "strobe"
  RT_CPU/3(b) -> Breaks/1
  d/1 -> RT_CPU/4(din)
  f_clk/1 -> precalculations/2(f_clk)
  mode/1 -> RT_CPU/3(mode)
  Data Type Conversion4/1 -> Counter_out(write_address)/1

== system uc3_preparation1_2017/CandHDL_hdl/hdlgenerate/FPGA_simulation ==
  M : Inport
  T : Inport  Port=2
  Cc0 : Inport  Port=3
  Cc1 : Inport  Port=4
  Cc2 : Inport  Port=5
  Count_out : Inport  Port=6
  we : Inport  Port=7
  " FPGA_Part" : Subsystem
  Gain : Gain  Gain=1/2^20  OutDataTypeStr=fixdt(1,32,19)
  Gain1 : Gain  Gain=1/2^20  OutDataTypeStr=fixdt(1,32,19)
  TimeGenerator : Subsystem
  y : Outport
  wires:
  T/1 -> Gain1/1
  M/1 -> Gain/1
  TimeGenerator/1(Time) -> " FPGA_Part"/6(Time)  "Time"
  Gain/1 -> TimeGenerator/1(M)
  Gain1/1 -> TimeGenerator/2(T)
  Cc0/1 -> " FPGA_Part"/1(Cc0)
  Cc1/1 -> " FPGA_Part"/2(Cc1)
  Cc2/1 -> " FPGA_Part"/3(Cc2)
  Count_out/1 -> " FPGA_Part"/4(Counter_out(write_addr))
  we/1 -> " FPGA_Part"/5(We(write_enable))
  TimeGenerator/2(read_add) -> " FPGA_Part"/7(read)
  " FPGA_Part"/1(output_wave(y)) -> y/1

== system uc3_preparation1_2017/CandHDL_hdl/hdlgenerate/Subsystem ==
  note: FPGA CONNECTIONS
  shared_signals_in_sig2 : Inport  OutDataTypeStr=int32
  shared_signals_in_sig3 : Inport  Port=2  OutDataTypeStr=int32
  shared_signals_in_sig4 : Inport  Port=3  OutDataTypeStr=int32
  shared_signals_in_sig5 : Inport  Port=4  OutDataTypeStr=int32
  shared_signals_in_sig6 : Inport  Port=5  OutDataTypeStr=int32
  shared_signals_in_sig7 : Inport  Port=6  OutDataTypeStr=int32
  shared_signals_in_sig8 : Inport  Port=7  OutDataTypeStr=int32
  Dynamic_Calculations : Subsystem
  duty1 : Outport  OutDataTypeStr=uint16
  wires:
  shared_signals_in_sig3/1 -> Dynamic_Calculations/2(c1)
  shared_signals_in_sig5/1 -> Dynamic_Calculations/4(write)
  shared_signals_in_sig4/1 -> Dynamic_Calculations/3(c2)
  shared_signals_in_sig6/1 -> Dynamic_Calculations/5(writeAddr)
  shared_signals_in_sig2/1 -> Dynamic_Calculations/1(c0)
  shared_signals_in_sig7/1 -> Dynamic_Calculations/6(M)
  Dynamic_Calculations/1(y) -> duty1/1
  shared_signals_in_sig8/1 -> Dynamic_Calculations/7(T)

== system uc3_preparation1_2017/CandHDL_c/cgenerate/Static Calculations/Coefficient Sequencer ==
  note: COEFFICIENT SEQUENCER
  note: Generates coefficients in a sequenced manner to be written to memory
  cc : Inport
  breakpoints : Inport  Port=2
  In3 : Inport  Port=3
  Trigger : TriggerPort  VariantControl=Variant  PortDimensions=1
  Coefficient Selector : Subsystem
  Counter : Subsystem
  c0 : Outport
  c1 : Outport  Port=2
  c2 : Outport  Port=3
  write : Outport  Port=4
  writeAddr : Outport  Port=5
  wires:
  breakpoints/1 -> Counter/1(breakpoints)
  In3/1 -> Counter/2(Reset)
  cc/1 -> Coefficient Selector/1(coeff)
  Counter/1(count) -> writeAddr/1, Coefficient Selector/2(rowIndex)
  Counter/2(write) -> write/1, Coefficient Selector/3(write)
  Coefficient Selector/1(c0) -> c0/1
  Coefficient Selector/2(c1) -> c1/1
  Coefficient Selector/3(c2) -> c2/1

== system uc3_preparation1_2017/CandHDL_c/cgenerate/Static Calculations/DETECT CHANGE ==
  note: Detects Change in Input Parameters For the Continious Run System
  note: DETECT CHANGE
  A : Inport
  mode : Inport  Port=2
  Duty Cycle : Inport  Port=3
  Breakpoints : Inport  Port=4
  pOrder : Inport  Port=5
  f : Inport  Port=6
  Detect Change{,1..5} (6 alike) : simulink/Logic and Bit Operations/Detect Change  vinit=0  OutDataTypeStr=boolean
  OR : Logic  Operator=OR  Inputs=6  AllPortsSameDT=off  OutDataTypeStr=boolean
  detectChange : Outport
  wires:
  Detect Change3/1 -> OR/4
  mode/1 -> Detect Change2/1
  Detect Change5/1 -> OR/6
  Detect Change1/1 -> OR/2
  Breakpoints/1 -> Detect Change4/1
  pOrder/1 -> Detect Change5/1
  Detect Change4/1 -> OR/5
  Detect Change2/1 -> OR/3
  Detect Change/1 -> OR/1
  Duty Cycle/1 -> Detect Change3/1
  f/1 -> Detect Change1/1
  A/1 -> Detect Change/1
  OR/1 -> detectChange/1

== system uc3_preparation1_2017/CandHDL_c/cgenerate/Static Calculations/precalculations ==
  f : Inport
  f_clk : Inport  Port=2
  Display : Display
  Display1 : Display
  Math Function1 : Math  Operator=pow  SaturateOnIntegerOverflow=on
  Math Function2 : Math  Operator=reciprocal  SaturateOnIntegerOverflow=on
  cte2 : Constant  Value=2  SampleTime=-1
  f_in_fclk : Product  Inputs=*/
  f_in_fclk1 : Product  Inputs=**
  n : Constant  Value=7  SampleTime=-1
  M : Outport
  n_out : Outport  Port=2
  T : Outport  Port=3
  wires:
  cte2/1 -> Math Function1/1  "two"
  n/1 -> Math Function1/2, n_out/1  "n"
  Math Function1/1 -> f_in_fclk1/1  "precalc"
  Math Function2/1 -> T/1  "T"
  f_in_fclk1/1 -> M/1  "M"
  f_clk/1 -> f_in_fclk/2, Display1/1  "f_clk"
  f_in_fclk/1 -> f_in_fclk1/2  "f_norm"
  f/1 -> Math Function2/1, Display/1, f_in_fclk/1

== system uc3_preparation1_2017/CandHDL_c/cgenerate/Subsystem/Counter ==
  note: The output is 0 if the comparison is false, and 1 if it is true.
  note: C
  strobe1 : Inport
  Chart : Stateflow chart  TreatAsAtomicUnit=on
  Compare To Zero2 : simulink/Logic and Bit Operations/Compare To Zero  relop=~=  OutDataTypeStr=boolean
  Compare To Zero3 : simulink/Logic and Bit Operations/Compare To Zero  relop=~=  OutDataTypeStr=boolean
  Delay1 : Delay  DelayLength=1
  Scope7 : Scope  NumInputPorts=3
  Sum2 : Sum  Inputs=|++  OutDataTypeStr=single
  Sum3 : Sum  Inputs=|++  OutDataTypeStr=single
  write_en : Outport
  counter_out : Outport  Port=2
  wires:
  Compare To Zero2/1 -> Sum2/1
  Sum3/1 -> Compare To Zero2/1
  Delay1/1 -> Sum2/2, Sum3/2
  Sum2/1 -> Chart/1(strobe)
  Chart/1(counter) -> Scope7/1, counter_out/1, Scope7/3, Compare To Zero3/1, Delay1/1  "A"
  strobe1/1 -> Sum3/1
  Compare To Zero3/1 -> Scope7/2, write_en/1  "B"

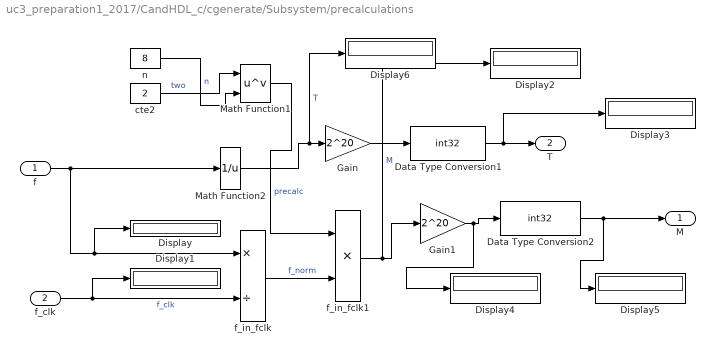
== system uc3_preparation1_2017/CandHDL_c/cgenerate/Subsystem/precalculations ==
  f : Inport
  f_clk : Inport  Port=2
  Data Type Conversion1 : DataTypeConversion  OutDataTypeStr=int32
  Data Type Conversion2 : DataTypeConversion  OutDataTypeStr=int32
  Display{,1..6} (7 alike) : Display
  Gain : Gain  Gain=2^20  OutDataTypeStr=single
  Gain1 : Gain  Gain=2^20  OutDataTypeStr=single
  Math Function1 : Math  Operator=pow  SaturateOnIntegerOverflow=on
  Math Function2 : Math  Operator=reciprocal  OutDataTypeStr=single  SaturateOnIntegerOverflow=on
  cte2 : Constant  Value=2  OutDataTypeStr=single  SampleTime=-1
  f_in_fclk : Product  Inputs=*/  OutDataTypeStr=single
  f_in_fclk1 : Product  Inputs=**  OutDataTypeStr=single
  n : Constant  Value=8  OutDataTypeStr=single  SampleTime=-1
  M : Outport
  T : Outport  Port=2
  wires:
  cte2/1 -> Math Function1/1  "two"
  n/1 -> Math Function1/2  "n"
  Math Function1/1 -> f_in_fclk1/1  "precalc"
  Math Function2/1 -> Display6/1, Gain/1  "T"
  f_clk/1 -> f_in_fclk/2, Display1/1  "f_clk"
  f_in_fclk/1 -> f_in_fclk1/2  "f_norm"
  f/1 -> Math Function2/1, Display/1, f_in_fclk/1
  Data Type Conversion1/1 -> Display3/1, T/1
  f_in_fclk1/1 -> Display2/1, Gain1/1  "M"
  Data Type Conversion2/1 -> Display5/1, M/1
  Gain/1 -> Data Type Conversion1/1
  Gain1/1 -> Display4/1, Data Type Conversion2/1

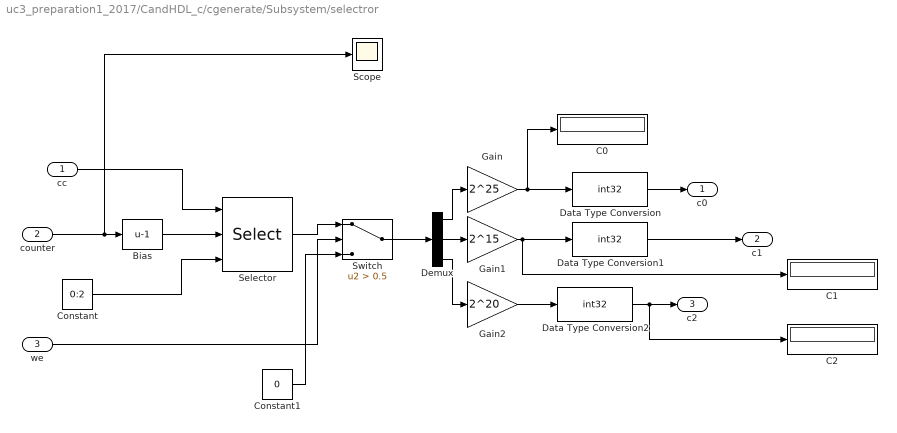
== system uc3_preparation1_2017/CandHDL_c/cgenerate/Subsystem/selectror ==
  cc : Inport
  counter : Inport  Port=2
  we : Inport  Port=3
  Bias : Bias  Bias=-1
  C0 : Display
  C1 : Display
  C2 : Display
  Constant : Constant  Value=0:2  OutDataTypeStr=single
  Constant1 : Constant  Value=0  OutDataTypeStr=single
  Data Type Conversion : DataTypeConversion  OutDataTypeStr=int32
  Data Type Conversion1 : DataTypeConversion  OutDataTypeStr=int32
  Data Type Conversion2 : DataTypeConversion  OutDataTypeStr=int32
  Demux : Demux  Outputs=3
  Gain : Gain  Gain=2^25  OutDataTypeStr=single
  Gain1 : Gain  Gain=2^15  OutDataTypeStr=single
  Gain2 : Gain  Gain=2^20  OutDataTypeStr=single
  Scope : Scope
  Selector : Selector  NumberOfDimensions=2  IndexMode=Zero-based  InputPortWidth=3  IndexOptions=Index vector (port),Index vector (port)  Indices=[1 3],1  OutputSizes=1,1
  Switch : Switch  Criteria=u2 > Threshold  Threshold=0.5  OutDataTypeStr=single
  c0 : Outport
  c1 : Outport  Port=2
  c2 : Outport  Port=3
  wires:
  cc/1 -> Selector/1
  Constant/1 -> Selector/3
  Data Type Conversion/1 -> c0/1
  Data Type Conversion1/1 -> c1/1
  Data Type Conversion2/1 -> C2/1, c2/1
  Gain/1 -> C0/1, Data Type Conversion/1
  Demux/1 -> Gain/1
  Gain1/1 -> Data Type Conversion1/1, C1/1
  Demux/2 -> Gain1/1
  Gain2/1 -> Data Type Conversion2/1
  Demux/3 -> Gain2/1
  counter/1 -> Bias/1, Scope/1
  Switch/1 -> Demux/1
  Selector/1 -> Switch/1
  we/1 -> Switch/2
  Constant1/1 -> Switch/3
  Bias/1 -> Selector/2

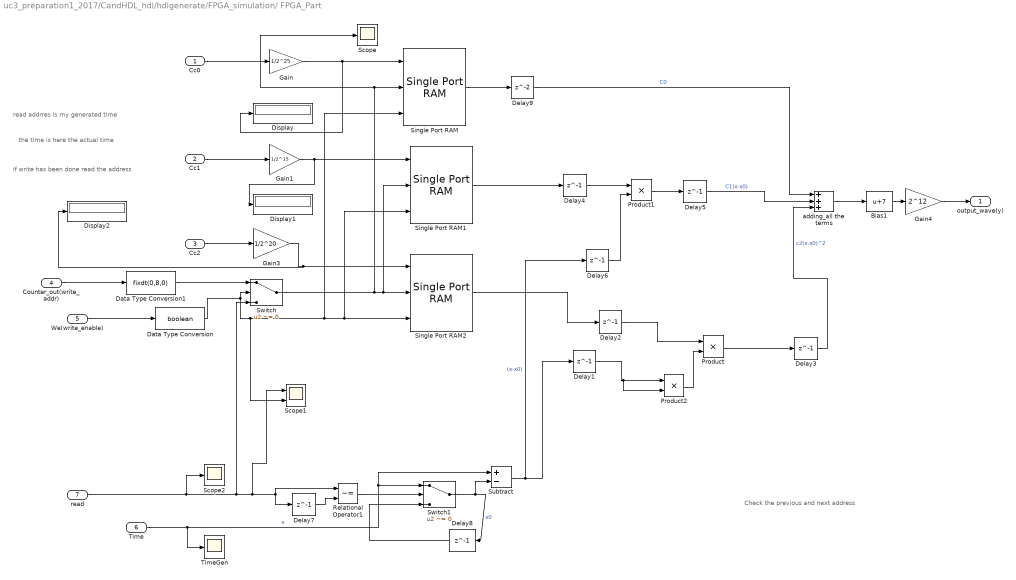
== system uc3_preparation1_2017/CandHDL_hdl/hdlgenerate/FPGA_simulation/ FPGA_Part ==
  note: Check the previous and next address
  note: if write has been done read the address
  note: the time is here the actual time
  note: read addrres is my generated time
  Cc0 : Inport
  Cc1 : Inport  Port=2
  Cc2 : Inport  Port=3
  Counter_out(write_addr) : Inport  Port=4
  We(write_enable) : Inport  Port=5
  Time : Inport  Port=6
  read : Inport  Port=7
  Bias1 : Bias  Bias=7
  Data Type Conversion : DataTypeConversion  OutDataTypeStr=boolean
  Data Type Conversion1 : DataTypeConversion  OutDataTypeStr=fixdt(0,8,0)
  Delay{1..8} (8 alike) : Delay  DelayLength=1
  Delay9 : Delay
  Display : Display
  Display1 : Display
  Display2 : Display
  Gain : Gain  Gain=1/2^25  OutDataTypeStr=fixdt(1,32,19)
  Gain1 : Gain  Gain=1/2^15  OutDataTypeStr=fixdt(1,32,19)
  Gain3 : Gain  Gain=1/2^20  OutDataTypeStr=fixdt(1,32,19)
  Gain4 : Gain  Gain=2^12  OutDataTypeStr=uint16
  Product : Product  OutDataTypeStr=fixdt(1,32,19)
  Product1 : Product  OutDataTypeStr=fixdt(1,32,19)
  Product2 : Product  OutDataTypeStr=fixdt(1,32,19)
  Relational Operator1 : RelationalOperator  Operator=~=  OutDataTypeStr=boolean  RndMeth=Simplest
  Scope : Scope
  Scope1 : Scope  NumInputPorts=2
  Scope2 : Scope
  Single Port RAM : hdlsllib/HDL RAMs/Single Port RAM  ram_size=8  dout_type=Old data
      settings: SourceProductName=HDL Coder  SourceProductBaseCode=HD
  Single Port RAM1 : hdlsllib/HDL RAMs/Single Port RAM  ram_size=8  dout_type=Old data
      settings: SourceProductName=HDL Coder  SourceProductBaseCode=HD
  Single Port RAM2 : hdlsllib/HDL RAMs/Single Port RAM  ram_size=8  dout_type=Old data
      settings: SourceProductName=HDL Coder  SourceProductBaseCode=HD
  Subtract : Sum  Inputs=+-  OutDataTypeStr=fixdt(1,32,19)
  Switch : Switch  Criteria=u2 ~= 0  OutDataTypeStr=fixdt(0,8,0)
  Switch1 : Switch  Criteria=u2 ~= 0  OutDataTypeStr=fixdt(1,32,19)
  TimeGen : Scope
  adding_all the terms : Sum  Inputs=+++  OutDataTypeStr=fixdt(1,32,19)
  output_wave(y) : Outport
  wires:
  Cc0/1 -> Gain/1
  Cc1/1 -> Gain1/1
  Cc2/1 -> Gain3/1
  Single Port RAM/1 -> Delay9/1
  We(write_enable)/1 -> Data Type Conversion/1
  Gain/1 -> Display/1, Single Port RAM/1
  Gain1/1 -> Display1/1, Single Port RAM1/1
  Gain3/1 -> Display2/1, Single Port RAM2/1
  Delay9/1 -> adding_all the terms/1  "C0"
  Delay2/1 -> Product/1
  Delay1/1 -> Product2/2, Product2/1
  Delay3/1 -> adding_all the terms/3  "c2(x-x0)^2"
  Delay4/1 -> Product1/1
  Product1/1 -> Delay5/1
  Delay5/1 -> adding_all the terms/2  "C1(x-x0)"
  Switch/1 -> Single Port RAM/2, Scope/1, Single Port RAM1/2, Single Port RAM2/2
  Data Type Conversion/1 -> Scope1/2, Single Port RAM1/3, Single Port RAM2/3, Single Port RAM/3, Switch/2
  Delay6/1 -> Product1/2
  Product2/1 -> Product/2
  Time/1 -> TimeGen/1, Switch1/1, Subtract/1  "x"
  Delay7/1 -> Relational Operator1/2
  Subtract/1 -> Delay6/1, Delay1/1  "(x-x0)"
  adding_all the terms/1 -> Bias1/1
  Switch1/1 -> Delay8/1, Subtract/2  "x0"
  Single Port RAM1/1 -> Delay4/1
  Single Port RAM2/1 -> Delay2/1
  Product/1 -> Delay3/1
  Relational Operator1/1 -> Switch1/2
  Delay8/1 -> Switch1/3
  read/1 -> Switch/3, Scope1/1, Relational Operator1/1, Delay7/1, Scope2/1
  Counter_out(write_addr)/1 -> Data Type Conversion1/1
  Data Type Conversion1/1 -> Switch/1
  Bias1/1 -> Gain4/1
  Gain4/1 -> output_wave(y)/1

== system uc3_preparation1_2017/CandHDL_hdl/hdlgenerate/FPGA_simulation/TimeGenerator ==
  M : Inport  OutDataTypeStr=fixdt(1,32,19)
  T : Inport  Port=2  OutDataTypeStr=fixdt(1,32,19)
  Add1 : Sum  OutDataTypeStr=fixdt(1,32,19)
  Bias : Bias  Bias=1
  Bit Slice : hdlsllib/Logic and Bit Operations/Bit Slice  lidx=26  ridx=19
  Constant1 : Constant  Value=0  OutDataTypeStr=fixdt(1,32,19)
  Constant2 : Constant  Value=2^(-8)  OutDataTypeStr=fixdt(1,32,19)
  Constant3 : Constant  Value=128  OutDataTypeStr=fixdt(1,32,19)
  Display{1..2,4..6} (5 alike) : Display
  Product : Product  OutDataTypeStr=fixdt(1,32,19)
  Product1 : Product  OutDataTypeStr=fixdt(1,32,19)
  Relational Operator : RelationalOperator  OutDataTypeStr=fixdt(1,32,19)  RndMeth=Nearest
  Switch : Switch  Threshold=0.5  OutDataTypeStr=fixdt(1,32,19)
  Unit Delay1 : UnitDelay  SampleTime=-1
  Time : Outport
  read_add : Outport  Port=2
  wires:
  Constant2/1 -> Product1/2
  Product/1 -> Time/1  "Time"
  Product1/1 -> Product/2
  Unit Delay1/1 -> Add1/2
  Constant1/1 -> Switch/1
  Relational Operator/1 -> Switch/2
  Add1/1 -> Display5/1, Switch/3, Display6/1, Relational Operator/1
  Constant3/1 -> Display1/1, Relational Operator/2
  M/1 -> Display2/1, Add1/1
  T/1 -> Product1/1
  Switch/1 -> Bit Slice/1, Unit Delay1/1, Product/1
  Bit Slice/1 -> Bias/1
  Bias/1 -> read_add/1, Display4/1

== system uc3_preparation1_2017/CandHDL_hdl/hdlgenerate/Subsystem/Dynamic_Calculations ==
  note: AWFG MODEL FPGA BLOCK
  c0 : Inport
  c1 : Inport  Port=2
  c2 : Inport  Port=3
  write : Inport  Port=4
  writeAddr : Inport  Port=5
  M : Inport  Port=6
  T : Inport  Port=7
  FPGA_Calculation : Subsystem
  Signal Scaling & Casting : Subsystem
  y : Outport
  wires:
  FPGA_Calculation/1(y) -> y/1
  c0/1 -> Signal Scaling & Casting/1(c0)
  c1/1 -> Signal Scaling & Casting/2(c1)
  c2/1 -> Signal Scaling & Casting/3(c2)
  write/1 -> Signal Scaling & Casting/4(write)
  writeAddr/1 -> Signal Scaling & Casting/5(writeAddr)
  T/1 -> Signal Scaling & Casting/7(T)
  Signal Scaling & Casting/6(Mi) -> FPGA_Calculation/6(M)
  Signal Scaling & Casting/7(Ti) -> FPGA_Calculation/7(T)
  Signal Scaling & Casting/5(writeAddri) -> FPGA_Calculation/5(writeAddr)
  Signal Scaling & Casting/4(writei) -> FPGA_Calculation/4(write)
  Signal Scaling & Casting/3(c2i) -> FPGA_Calculation/3(c2)
  Signal Scaling & Casting/2(c1i) -> FPGA_Calculation/2(c1)
  Signal Scaling & Casting/1(c0i) -> FPGA_Calculation/1(c0)
  M/1 -> Signal Scaling & Casting/6(M)

== system uc3_preparation1_2017/CandHDL_c/cgenerate/Static Calculations/Coefficient Sequencer/Coefficient Selector ==
  note: COEFFICIENT SELECTOR
  note: Selects a single row from the coefficients matrix based on the counter value
  coeff : Inport
  rowIndex : Inport  Port=2
  write : Inport  Port=3
  Constant : Constant  Value=[0:2]
  Demux : Demux  Outputs=3
  Selector : Selector  NumberOfDimensions=2  IndexMode=Zero-based  InputPortWidth=3  IndexOptions=Starting index (port),Index vector (port)  Indices=[1 3],[0 : 2]  OutputSizes=1,1
  Switch1 : Switch  Criteria=u2 ~= 0
  c0 : Outport
  c1 : Outport  Port=2
  c2 : Outport  Port=3
  wires:
  rowIndex/1 -> Selector/2
  coeff/1 -> Selector/1
  Selector/1 -> Switch1/1
  Demux/3 -> c2/1
  write/1 -> Switch1/2, Switch1/3
  Demux/2 -> c1/1
  Demux/1 -> c0/1
  Constant/1 -> Selector/3
  Switch1/1 -> Demux/1

== system uc3_preparation1_2017/CandHDL_c/cgenerate/Static Calculations/Coefficient Sequencer/Counter ==
  note: This Block counts on every clock tick up to the number of breakpoints
  note: COUNTER BLOCK
  breakpoints : Inport
  Reset : Inport  Port=2
  Counter : dspswit3/Counter  Direction=Up  CountEvent=Non-zero sample  CounterSize=User defined  MaxCount=255  InitialCount=0  Output=Count  HitValue=32  ResetInput=on  SamplesPerFrame=1  Ts=1  CntDtype=single  HitDtype=Logical
  Delay : Delay  DelayLength=1
  GreaterThan : RelationalOperator  Operator=>  OutDataTypeStr=boolean  RndMeth=Simplest
  count : Outport
  write : Outport  Port=2
  wires:
  GreaterThan/1 -> write/1, Counter/1
  Counter/1 -> count/1, Delay/1
  breakpoints/1 -> GreaterThan/1
  Delay/1 -> GreaterThan/2
  Reset/1 -> Counter/2

== system uc3_preparation1_2017/CandHDL_hdl/hdlgenerate/Subsystem/Dynamic_Calculations/FPGA_Calculation ==
  note: AWFG DYNAMIC CALCULATIONS
  note: This block will run on FPGA, responsible for calculating polynomial
  c0 : Inport
  c1 : Inport  Port=2
  c2 : Inport  Port=3
  write : Inport  Port=4
  writeAddr : Inport  Port=5
  M : Inport  Port=6
  T : Inport  Port=7
  Polynomial_Calculation : Subsystem
  TimeGenerator : Subsystem
  Write_to_Memory : Subsystem
  y : Outport
  wires:
  c1/1 -> Write_to_Memory/3(c1)
  c0/1 -> Write_to_Memory/2(c0)
  Polynomial_Calculation/1(y) -> y/1
  c2/1 -> Write_to_Memory/4(c2)
  T/1 -> TimeGenerator/2(T)
  Write_to_Memory/1(c0Ram) -> Polynomial_Calculation/3(c0Ram)
  TimeGenerator/2(readAddr) -> Write_to_Memory/1(readAddr), Polynomial_Calculation/2(breakpoints)
  M/1 -> TimeGenerator/1(M)
  Write_to_Memory/3(c2Ram) -> Polynomial_Calculation/5(c2Ram)
  write/1 -> Write_to_Memory/5(write)
  writeAddr/1 -> Write_to_Memory/6(writeAddr)
  Write_to_Memory/2(c1Ram) -> Polynomial_Calculation/4(c1Ram)
  TimeGenerator/1(Time) -> Polynomial_Calculation/1(Time)

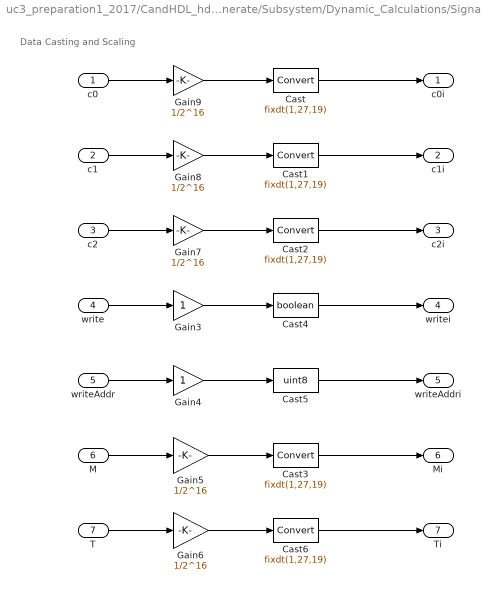
== system uc3_preparation1_2017/CandHDL_hdl/hdlgenerate/Subsystem/Dynamic_Calculations/Signal Scaling & Casting ==
  note: Data Casting and Scaling
  c0 : Inport
  c1 : Inport  Port=2
  c2 : Inport  Port=3
  write : Inport  Port=4
  writeAddr : Inport  Port=5
  M : Inport  Port=6
  T : Inport  Port=7
  Cast{,1..3,6} (5 alike) : DataTypeConversion  OutDataTypeStr=fixdt(1,27,19)
  Cast4 : DataTypeConversion  OutDataTypeStr=boolean
  Cast5 : DataTypeConversion  OutDataTypeStr=uint8
  Gain3 : Gain
  Gain4 : Gain
  Gain{5..9} (5 alike) : Gain  Gain=1/2^16
  c0i : Outport
  c1i : Outport  Port=2
  c2i : Outport  Port=3
  writei : Outport  Port=4
  writeAddri : Outport  Port=5
  Mi : Outport  Port=6
  Ti : Outport  Port=7
  wires:
  c0/1 -> Gain9/1
  c1/1 -> Gain8/1
  c2/1 -> Gain7/1
  write/1 -> Gain3/1
  writeAddr/1 -> Gain4/1
  M/1 -> Gain5/1
  T/1 -> Gain6/1
  Gain9/1 -> Cast/1
  Gain8/1 -> Cast1/1
  Gain7/1 -> Cast2/1
  Gain3/1 -> Cast4/1
  Gain4/1 -> Cast5/1
  Gain5/1 -> Cast3/1
  Gain6/1 -> Cast6/1
  Cast6/1 -> Ti/1
  Cast5/1 -> writeAddri/1
  Cast4/1 -> writei/1
  Cast2/1 -> c2i/1
  Cast1/1 -> c1i/1
  Cast/1 -> c0i/1
  Cast3/1 -> Mi/1

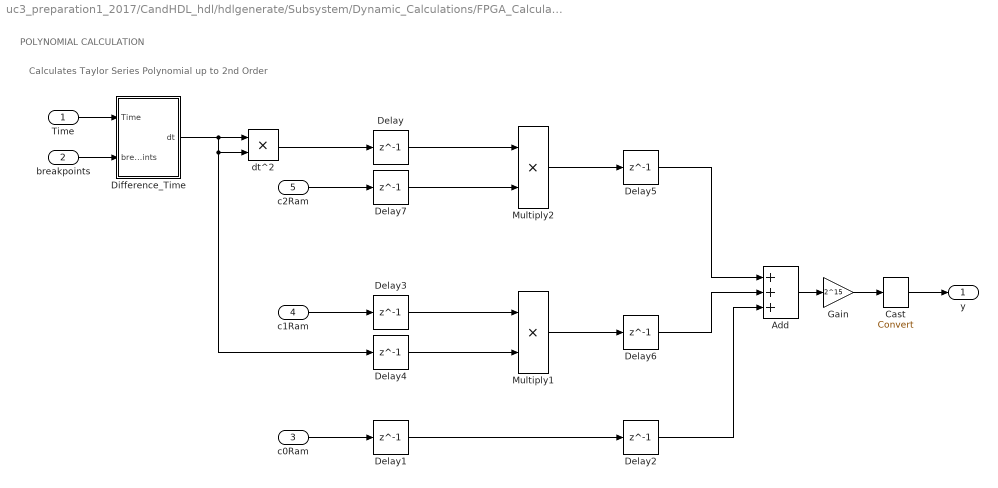
== system uc3_preparation1_2017/CandHDL_hdl/hdlgenerate/Subsystem/Dynamic_Calculations/FPGA_Calculation/Polynomial_Calculation ==
  note: POLYNOMIAL CALCULATION
  note: Calculates Taylor Series Polynomial up to 2nd Order
  Time : Inport
  breakpoints : Inport  Port=2
  c0Ram : Inport  Port=3
  c1Ram : Inport  Port=4
  c2Ram : Inport  Port=5
  Add : Sum  Inputs=3  OutDataTypeStr=fixdt(1,27,19)
  Cast : DataTypeConversion
  Delay{,1..7} (8 alike) : Delay  DelayLength=1
  Difference_Time : Subsystem
  Gain : Gain  Gain=2^15
  Multiply1 : Product  OutDataTypeStr=fixdt(1,27,19)
  Multiply2 : Product  OutDataTypeStr=fixdt(1,27,19)  InputSameDT=on
  dt^2 : Product  OutDataTypeStr=fixdt(1,27,19)
  y : Outport
  wires:
  dt^2/1 -> Delay/1
  c0Ram/1 -> Delay1/1
  Delay1/1 -> Delay2/1
  c1Ram/1 -> Delay3/1
  Delay3/1 -> Multiply1/1
  Delay4/1 -> Multiply1/2
  c2Ram/1 -> Delay7/1
  Delay/1 -> Multiply2/1
  Multiply1/1 -> Delay6/1
  Multiply2/1 -> Delay5/1
  Delay7/1 -> Multiply2/2
  Delay5/1 -> Add/1
  Delay6/1 -> Add/2
  Delay2/1 -> Add/3
  Difference_Time/1(dt) -> dt^2/1, dt^2/2, Delay4/1
  Time/1 -> Difference_Time/1(Time)
  breakpoints/1 -> Difference_Time/2(breakpoints)
  Add/1 -> Gain/1
  Gain/1 -> Cast/1
  Cast/1 -> y/1

== system uc3_preparation1_2017/CandHDL_hdl/hdlgenerate/Subsystem/Dynamic_Calculations/FPGA_Calculation/TimeGenerator ==
  note: TIME GENERATOR & ACCUMULATOR
  M : Inport
  T : Inport  Port=2
  Add1 : Sum  OutDataTypeStr=fixdt(0,26,19)
  Bias : Bias  Bias=1
  Bit Slice : hdlsllib/Logic and Bit Operations/Bit Slice  lidx=26  ridx=19
  Cast : DataTypeConversion  OutDataTypeStr=fixdt(1,27,19)
  Constant2 : Constant  Value=2^-7  OutDataTypeStr=fixdt(1,27,19)
  Delay : Delay  DelayLength=1
  Product : Product  OutDataTypeStr=fixdt(1,27,19)
  Product1 : Product  OutDataTypeStr=fixdt(1,27,19)
  Time : Outport
  readAddr : Outport  Port=2
  wires:
  Product/1 -> Time/1  "Time"
  Product1/1 -> Product/2
  Add1/1 -> Cast/1
  Bit Slice/1 -> Bias/1
  M/1 -> Add1/2
  T/1 -> Product1/1
  Delay/1 -> Add1/1
  Cast/1 -> Bit Slice/1, Product/1, Delay/1
  Bias/1 -> readAddr/1
  Constant2/1 -> Product1/2
